simulink model "fboard_xaui"  (Simulink 6.2)
settings: Solver=FixedStepDiscrete  SolverMode=SingleTasking  StartTime=0.0  StopTime=10.0  FixedStep=1  RelTol=1e-3
libraries: xbsIndex_r3 x338, fb_xaui x1, newfft_library x1
(part 2 of 3)

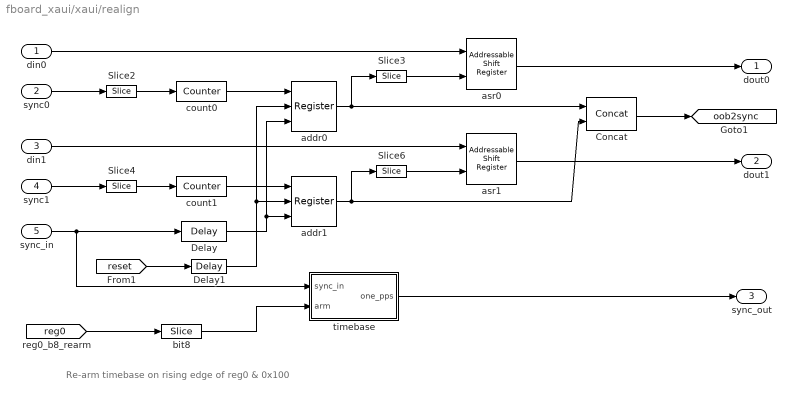
== system fboard_xaui/xaui/realign ==
  note: Re-arm timebase on rising
      | edge of reg0 & 0x100
  din0 : Inport  Port=1  LatchInput=off
  sync0 : Inport  Port=2  LatchInput=off
  din1 : Inport  Port=3  LatchInput=off
  sync1 : Inport  Port=4  LatchInput=off
  sync_in : Inport  Port=5  LatchInput=off
  Concat : xbsIndex_r3/Concat  num_inputs=2  explicit_period=off  period=1  dbl_ovrd=off
  Delay : xbsIndex_r3/Delay  latency=1  reg_retiming=off  explicit_period=off  period=1  en=off  accept_only_valid=off  init_zero=on  dbl_ovrd=off  show_param=off
      settings: xl_area=[1 1 0 0 0 0 0]
  Delay1 : xbsIndex_r3/Delay  latency=1  reg_retiming=off  explicit_period=off  period=1  en=off  accept_only_valid=off  init_zero=on  dbl_ovrd=off  show_param=off
      settings: xl_area=[1 1 0 0 0 0 0]
  Slice2 : xbsIndex_r3/Slice  mode=Lower Bit Location + Width  nbits=1  bit1=0  base1=MSB of Input  bit0=0  base0=LSB of Input  boolean_output=on  explicit_period=off  period=1  dbl_ovrd=off
  Slice3 : xbsIndex_r3/Slice  mode=Lower Bit Location + Width  nbits=6  bit1=0  base1=MSB of Input  bit0=0  base0=LSB of Input  boolean_output=off  explicit_period=off  period=1  dbl_ovrd=off
  Slice4 : xbsIndex_r3/Slice  mode=Lower Bit Location + Width  nbits=1  bit1=0  base1=MSB of Input  bit0=0  base0=LSB of Input  boolean_output=on  explicit_period=off  period=1  dbl_ovrd=off
  Slice6 : xbsIndex_r3/Slice  mode=Lower Bit Location + Width  nbits=6  bit1=0  base1=MSB of Input  bit0=0  base0=LSB of Input  boolean_output=off  explicit_period=off  period=1  dbl_ovrd=off
  addr0 : xbsIndex_r3/Register  init=hex2dec('DEC0')  reg_only_valid=off  explicit_period=off  period=1  rst=on  en=on  out_en=off  dbl_ovrd=off  show_param=on
      settings: xl_area=[3 6 0 0 0 0 0]
  addr1 : xbsIndex_r3/Register  init=hex2dec('DEC0')  reg_only_valid=off  explicit_period=off  period=1  rst=on  en=on  out_en=off  dbl_ovrd=off  show_param=on
      settings: xl_area=[3 6 0 0 0 0 0]
  asr0 : xbsIndex_r3/Addressable Shift Register  infer_latency=on  depth=64  initVector=[0]  explicit_period=off  period=1  accept_only_valid=off  en=off  dbl_ovrd=off  show_param=on  use_rpm=on  gen_core=off
      settings: xl_area=[192 0 0 384 0 0 0]
  asr1 : xbsIndex_r3/Addressable Shift Register  infer_latency=on  depth=64  initVector=[0]  explicit_period=off  period=1  accept_only_valid=off  en=off  dbl_ovrd=off  show_param=on  use_rpm=on  gen_core=off
      settings: xl_area=[192 0 0 384 0 0 0]
  bit8 : xbsIndex_r3/Slice  mode=Lower Bit Location + Width  nbits=1  bit1=12  base1=MSB of Input  bit0=8  base0=LSB of Input  boolean_output=on  explicit_period=off  period=1  dbl_ovrd=off
  count0 : xbsIndex_r3/Counter  cnt_type=Count Limited  n_bits=16  bin_pt=0  arith_type=Unsigned  start_count=0  cnt_to=hex2dec('FFFF')  cnt_by_val=1  operation=Up  explicit_period=off  period=1  load_pin=off  rst=on  en=off  dbl_ovrd=off  show_param=on  use_rpm=on  gen_core=off
      settings: xl_area=[3 6 0 6 0 0 0]
  count1 : xbsIndex_r3/Counter  cnt_type=Count Limited  n_bits=16  bin_pt=0  arith_type=Unsigned  start_count=0  cnt_to=hex2dec('FFFF')  cnt_by_val=1  operation=Up  explicit_period=off  period=1  load_pin=off  rst=on  en=off  dbl_ovrd=off  show_param=on  use_rpm=on  gen_core=off
      settings: xl_area=[3 6 0 6 0 0 0]
  timebase : Subsystem
  dout0 : Outport
  dout1 : Outport  Port=2
  sync_out : Outport  Port=3
  tag scope: oob2sync=global
  wires:
  count0/1 -> addr0/1
  addr0/1 -> Slice3/1, Concat/1
  count1/1 -> addr1/1
  addr1/1 -> Slice6/1, Concat/2
  din0/1 -> asr0/1
  asr0/1 -> dout0/1
  sync0/1 -> Slice2/1
  din1/1 -> asr1/1
  asr1/1 -> dout1/1
  sync1/1 -> Slice4/1
  sync_in/1 -> Delay/1, timebase/1(sync_in)
  timebase/1(one_pps) -> sync_out/1
  bit8/1 -> timebase/2(arm)
  [reg0] -> bit8/1
  Slice2/1 -> count0/1
  Slice4/1 -> count1/1
  Delay/1 -> addr0/3, addr1/3
  Slice3/1 -> asr0/2
  Slice6/1 -> asr1/2
  Concat/1 -> [oob2sync]
  [reset] -> Delay1/1
  Delay1/1 -> addr0/2, addr1/2

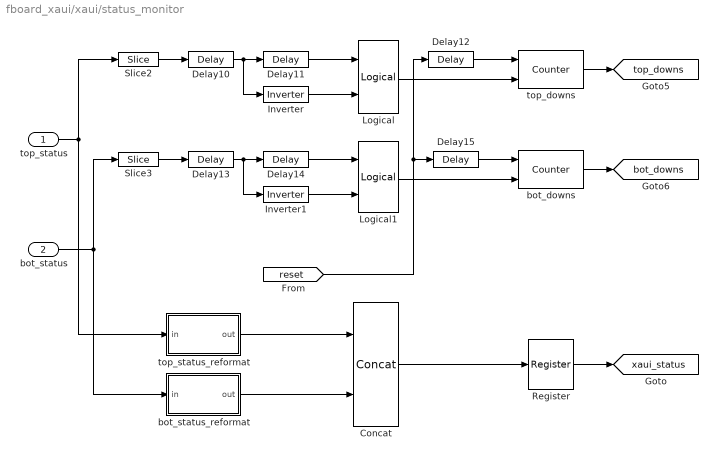
== system fboard_xaui/xaui/status_monitor ==
  top_status : Inport  Port=1  LatchInput=off
  bot_status : Inport  Port=2  LatchInput=off
  Concat : xbsIndex_r3/Concat  num_inputs=2  explicit_period=off  period=1  dbl_ovrd=off
  Delay{10..15} (6 alike) : xbsIndex_r3/Delay  latency=1  reg_retiming=off  explicit_period=off  period=1  en=off  accept_only_valid=off  init_zero=on  dbl_ovrd=off  show_param=off
      settings: xl_area=[0, 0, 0, 0, 0, 0, 0]
  Inverter : xbsIndex_r3/Inverter  latency=0  explicit_period=off  period=1  en=off  dbl_ovrd=off  show_param=off
      settings: xl_area=[0, 0, 0, 0, 0, 0, 0]
  Inverter1 : xbsIndex_r3/Inverter  latency=0  explicit_period=off  period=1  en=off  dbl_ovrd=off  show_param=off
      settings: xl_area=[0, 0, 0, 0, 0, 0, 0]
  Logical : xbsIndex_r3/Logical  logical_function=AND  inputs=2  precision=Full  arith_type=Unsigned  n_bits=8  bin_pt=2  align_bp=on  latency=0  explicit_period=off  period=1  en=off  dbl_ovrd=off  show_param=off
      settings: xl_area=[0, 0, 0, 0, 0, 0, 0]
  Logical1 : xbsIndex_r3/Logical  logical_function=AND  inputs=2  precision=Full  arith_type=Unsigned  n_bits=8  bin_pt=2  align_bp=on  latency=0  explicit_period=off  period=1  en=off  dbl_ovrd=off  show_param=off
      settings: xl_area=[0, 0, 0, 0, 0, 0, 0]
  Register : xbsIndex_r3/Register  init=0  reg_only_valid=off  explicit_period=off  period=1  rst=off  en=off  out_en=off  dbl_ovrd=off  show_param=off
      settings: xl_area=[0, 0, 0, 0, 0, 0, 0]
  Slice2 : xbsIndex_r3/Slice  mode=Lower Bit Location + Width  nbits=1  bit1=12  base1=MSB of Input  bit0=12  base0=LSB of Input  boolean_output=on  explicit_period=off  period=1  dbl_ovrd=off
  Slice3 : xbsIndex_r3/Slice  mode=Lower Bit Location + Width  nbits=1  bit1=12  base1=MSB of Input  bit0=12  base0=LSB of Input  boolean_output=on  explicit_period=off  period=1  dbl_ovrd=off
  bot_downs : xbsIndex_r3/Counter  cnt_type=Free Running  n_bits=32  bin_pt=0  arith_type=Unsigned  start_count=0  cnt_to=Inf  cnt_by_val=1  operation=Up  explicit_period=off  period=1  load_pin=off  rst=on  en=on  dbl_ovrd=off  show_param=off  use_rpm=on  gen_core=off
      settings: xl_area=[0, 0, 0, 0, 0, 0, 0]
  bot_status_reformat : Subsystem
  top_downs : xbsIndex_r3/Counter  cnt_type=Free Running  n_bits=32  bin_pt=0  arith_type=Unsigned  start_count=0  cnt_to=Inf  cnt_by_val=1  operation=Up  explicit_period=off  period=1  load_pin=off  rst=on  en=on  dbl_ovrd=off  show_param=off  use_rpm=on  gen_core=off
      settings: xl_area=[0, 0, 0, 0, 0, 0, 0]
  top_status_reformat : Subsystem
  tag scope: bot_downs=global, top_downs=global, xaui_status=global
  wires:
  top_status/1 -> Slice2/1, top_status_reformat/1(in)
  bot_status/1 -> Slice3/1, bot_status_reformat/1(in)
  top_status_reformat/1(out) -> Concat/1
  bot_status_reformat/1(out) -> Concat/2
  Register/1 -> [xaui_status]
  Concat/1 -> Register/1
  [reset] -> Delay15/1, Delay12/1
  Delay10/1 -> Delay11/1, Inverter/1
  Delay11/1 -> Logical/1
  Inverter/1 -> Logical/2
  Delay12/1 -> top_downs/1
  top_downs/1 -> [top_downs]
  Delay13/1 -> Delay14/1, Inverter1/1
  Delay14/1 -> Logical1/1
  Inverter1/1 -> Logical1/2
  Delay15/1 -> bot_downs/1
  bot_downs/1 -> [bot_downs]
  Logical1/1 -> bot_downs/2
  Logical/1 -> top_downs/2
  Slice2/1 -> Delay10/1
  Slice3/1 -> Delay13/1

== system fboard_xaui/xaui/sync_monitor ==
  top_sync : Inport  Port=1  LatchInput=off
  bot_sync : Inport  Port=2  LatchInput=off
  Delay{4..7} (4 alike) : xbsIndex_r3/Delay  latency=1  reg_retiming=off  explicit_period=off  period=1  en=off  accept_only_valid=off  init_zero=on  dbl_ovrd=off  show_param=off
      settings: xl_area=[0, 0, 0, 0, 0, 0, 0]
  Slice : xbsIndex_r3/Slice  mode=Lower Bit Location + Width  nbits=1  bit1=0  base1=MSB of Input  bit0=0  base0=LSB of Input  boolean_output=on  explicit_period=off  period=1  dbl_ovrd=off
  Slice1 : xbsIndex_r3/Slice  mode=Lower Bit Location + Width  nbits=1  bit1=0  base1=MSB of Input  bit0=0  base0=LSB of Input  boolean_output=on  explicit_period=off  period=1  dbl_ovrd=off
  bot_syncs : xbsIndex_r3/Counter  cnt_type=Free Running  n_bits=32  bin_pt=0  arith_type=Unsigned  start_count=0  cnt_to=Inf  cnt_by_val=1  operation=Up  explicit_period=off  period=1  load_pin=off  rst=on  en=on  dbl_ovrd=off  show_param=off  use_rpm=on  gen_core=off
      settings: xl_area=[0, 0, 0, 0, 0, 0, 0]
  top_syncs : xbsIndex_r3/Counter  cnt_type=Free Running  n_bits=32  bin_pt=0  arith_type=Unsigned  start_count=0  cnt_to=Inf  cnt_by_val=1  operation=Up  explicit_period=off  period=1  load_pin=off  rst=on  en=on  dbl_ovrd=off  show_param=off  use_rpm=on  gen_core=off
      settings: xl_area=[0, 0, 0, 0, 0, 0, 0]
  tag scope: bot_syncs=global, top_syncs=global
  wires:
  bot_sync/1 -> Slice1/1
  Delay4/1 -> top_syncs/1
  Delay5/1 -> bot_syncs/1
  top_syncs/1 -> [top_syncs]
  bot_syncs/1 -> [bot_syncs]
  Delay6/1 -> top_syncs/2
  Delay7/1 -> bot_syncs/2
  top_sync/1 -> Slice/1
  [reset] -> Delay5/1, Delay4/1
  Slice1/1 -> Delay7/1
  Slice/1 -> Delay6/1

== system fboard_xaui/xaui/sync_sel ==
  note: reg0 & 0x30
  top_sync : Inport  Port=1  LatchInput=off
  bot_sync : Inport  Port=2  LatchInput=off
  ext_sync : Inport  Port=3  LatchInput=off
  Delay : xbsIndex_r3/Delay  latency=31  reg_retiming=off  explicit_period=off  period=1  en=off  accept_only_valid=off  init_zero=on  dbl_ovrd=off  show_param=off
      settings: xl_area=[0, 0, 0, 0, 0, 0, 0]
  Mux : xbsIndex_r3/Mux  inputs=4  precision=Full  arith_type="Signed  (2's comp)"  n_bits=8  bin_pt=2  quantization=Truncate  overflow=Wrap  latency=1  explicit_period=off  period=1  en=off  dbl_ovrd=off  show_param=off  mux_type=off  use_rpm=off  gen_core=off
      settings: xl_area=[0, 0, 0, 0, 0, 0, 0]
  Slice1 : xbsIndex_r3/Slice  mode=Lower Bit Location + Width  nbits=1  bit1=0  base1=MSB of Input  bit0=1  base0=LSB of Input  boolean_output=on  explicit_period=off  period=1  dbl_ovrd=off
  Slice4 : xbsIndex_r3/Slice  mode=Lower Bit Location + Width  nbits=1  bit1=0  base1=MSB of Input  bit0=1  base0=LSB of Input  boolean_output=on  explicit_period=off  period=1  dbl_ovrd=off
  b5_b4 : xbsIndex_r3/Slice  mode=Lower Bit Location + Width  nbits=2  bit1=12  base1=MSB of Input  bit0=4  base0=LSB of Input  boolean_output=off  explicit_period=off  period=1  dbl_ovrd=off
  sync_out : Outport
  wires:
  Mux/1 -> Delay/1
  top_sync/1 -> Slice4/1
  bot_sync/1 -> Slice1/1
  Delay/1 -> sync_out/1
  b5_b4/1 -> Mux/1
  [reg0] -> b5_b4/1
  ext_sync/1 -> Mux/4, Mux/5
  Slice4/1 -> Mux/2
  Slice1/1 -> Mux/3

== system fboard_xaui/xaui/uflow_monitor ==
  note: Count rising edges of the rx_empty signals
  top_rx_empty : Inport  Port=1  LatchInput=off
  bot_rx_empty : Inport  Port=2  LatchInput=off
  Concat : xbsIndex_r3/Concat  num_inputs=2  explicit_period=off  period=1  dbl_ovrd=off
  Delay{1,11..12,15} (4 alike) : xbsIndex_r3/Delay  latency=1  reg_retiming=off  explicit_period=off  period=1  en=off  accept_only_valid=off  init_zero=on  dbl_ovrd=off  show_param=off
      settings: xl_area=[0, 0, 0, 0, 0, 0, 0]
  Expression : xbsIndex_r3/Expression  expression=curr & ~prev  precision=Full  arith_type=Unsigned  n_bits=8  bin_pt=2  align_bp=on  latency=0  explicit_period=off  period=1  en=off  dbl_ovrd=off  show_param=off
      settings: xl_area=[0, 0, 0, 0, 0, 0, 0]
  Expression1 : xbsIndex_r3/Expression  expression=curr & ~prev  precision=Full  arith_type=Unsigned  n_bits=8  bin_pt=2  align_bp=on  latency=0  explicit_period=off  period=1  en=off  dbl_ovrd=off  show_param=off
      settings: xl_area=[0, 0, 0, 0, 0, 0, 0]
  bot_uflows : xbsIndex_r3/Counter  cnt_type=Free Running  n_bits=16  bin_pt=0  arith_type=Unsigned  start_count=0  cnt_to=Inf  cnt_by_val=1  operation=Up  explicit_period=off  period=1  load_pin=off  rst=on  en=on  dbl_ovrd=off  show_param=off  use_rpm=on  gen_core=off
      settings: xl_area=[0, 0, 0, 0, 0, 0, 0]
  top_uflows : xbsIndex_r3/Counter  cnt_type=Free Running  n_bits=16  bin_pt=0  arith_type=Unsigned  start_count=0  cnt_to=Inf  cnt_by_val=1  operation=Up  explicit_period=off  period=1  load_pin=off  rst=on  en=on  dbl_ovrd=off  show_param=off  use_rpm=on  gen_core=off
      settings: xl_area=[0, 0, 0, 0, 0, 0, 0]
  tag scope: xaui_uflows=global
  wires:
  [reset] -> Delay15/1, Delay12/1
  Delay12/1 -> top_uflows/1
  top_uflows/1 -> Concat/1
  Delay15/1 -> bot_uflows/1
  bot_uflows/1 -> Concat/2
  Concat/1 -> [xaui_uflows]
  Delay11/1 -> Expression/2
  top_rx_empty/1 -> Delay11/1, Expression/1
  Expression/1 -> top_uflows/2
  Delay1/1 -> Expression1/2
  bot_rx_empty/1 -> Expression1/1, Delay1/1
  Expression1/1 -> bot_uflows/2

== system fboard_xaui/zbt_transpose/dvgen ==
  note: This dvgen block generates a dv signal based on sync_in's rising
      | edge and the value of ds_sel (downsample select), which is taken
      | from a global goto tag.  ds_sel can range from 0 to 7.  The dv
      | signal will be asserted for one cycle every 2^ds_sel cycles starting
      | with the first cycle after sync_out's rising edge.  Note that sync_in
      | may be one or many cycles wide, but it should probably be no
      | wider than 2^ds_sel cycles for typical usage.  sync_out is always
      | one cycle wide (corresponding to the first active cycle of sync_in).
  note: == Example Timing Diagrams ==
      |
      | -------  ds_sel == 0  -------
      | sync_in : .S................
      | sync_out : ....S.............
      | dv : 111111111111111111
      |
      | -------  ds_sel == 1  -------
      | sync_in : .S................
      | sync_out : ....S.............
      | dv : XXXX1.1.1.1.1.1.1.
      |
      | -------  ds_sel == 2  -------
      | sync_in : .SSSS.............
      | sync_out : ....S.............
      | dv : XXXX1...1...1...1.
  note: Only honor new ds_sel value
      | on rising edge of sync_in
  sync_in : Inport  Port=1  LatchInput=off
  Constant2 : xbsIndex_r3/Constant  const=0  equ=P=C  arith_type=Unsigned  n_bits=1  bin_pt=0  opselect=C  inp2=PCIN>>17  opr=+  inp1=P  carry=CIN  iostate=0  explicit_period=on  period=1  dbl_ovrd=off
  Counter : xbsIndex_r3/Counter  cnt_type=Free Running  n_bits=7  bin_pt=0  arith_type=Unsigned  start_count=0  cnt_to=Inf  cnt_by_val=1  operation=Up  explicit_period=off  period=1  load_pin=off  rst=on  en=off  dbl_ovrd=off  show_param=on  use_rpm=on  gen_core=off
      settings: xl_area=[0, 0, 0, 0, 0, 0, 0]
  Delay : xbsIndex_r3/Delay  latency=3  reg_retiming=off  explicit_period=off  period=1  en=off  accept_only_valid=off  init_zero=on  dbl_ovrd=off  show_param=off
      settings: xl_area=[0, 0, 0, 0, 0, 0, 0]
  Mux : xbsIndex_r3/Mux  inputs=8  precision=Full  arith_type="Signed  (2's comp)"  n_bits=8  bin_pt=2  quantization=Truncate  overflow=Wrap  latency=1  explicit_period=off  period=1  en=off  dbl_ovrd=off  show_param=off  mux_type=off  use_rpm=off  gen_core=off
      settings: xl_area=[0, 0, 0, 0, 0, 0, 0]
  Register2 : xbsIndex_r3/Register  init=0  reg_only_valid=off  explicit_period=off  period=1  rst=off  en=on  out_en=off  dbl_ovrd=off  show_param=off
      settings: xl_area=[0, 0, 0, 0, 0, 0, 0]
  Relational : xbsIndex_r3/Relational  mode=a=b  latency=1  explicit_period=off  period=1  en=off  dbl_ovrd=off  show_param=on
      settings: xl_area=[0, 0, 0, 0, 0, 0, 0]
  bit_slicer : Subsystem
  edge_detect : Subsystem  mask(Edge Detector){edge=Rising, polarity=Active High, xin=floor([0.5:0.5:5])*0.08, yin={[-1,-1,1,1,1,1,1,1,1,1],[1,1,-1,-1,-1,-1,-1,-1,-1,-1],[-1,-1,1,1,1,1,-1,-1,-1,-1]}, xout=1-floor([5:-0.5:0.5])*0.08, yout={[-1,-1,1,1,-1,-1,-1,-1,-1,-1],[-1,-1,1,1,-1,-1,-1,-1,-1,-1],[-1,-1,1,1,-1,-1,1,1,-1,-1]}}
      mask prompts: edge "Edge Type"; polarity "Output Polarity"; xin "Input X Positions"; yin "Input Y Positions"; xout "Output X Positions"; yout "Output Y Positions"
      mask help: Output is active for one-cycle after each edge of the specified type (i.e. rising, falling or both).
      mask init:
      | edge_detect_init(gcb,edge,polarity);
      settings: AttributesFormatString=|
      | rising edge
      | active high
      mask Help: Output is active for one-cycle after each edge of the specified type (i.e. rising, falling, or both).  Latency is zero.
      mask StyleString: popup(Rising|Falling|Both),popup(Active High|Active Low),edit,edit,edit,edit
      mask Display:
      | plot(xin,0.5+yin{edge}*0.2)
      | plot(xout,0.5+yout{edge}*0.2*(3-2*polarity))
  sync_out : Outport
  dv : Outport  Port=2
  wires:
  bit_slicer/1(zero) -> Mux/2
  bit_slicer/2(b0_0) -> Mux/3
  bit_slicer/3(b1_0) -> Mux/4
  bit_slicer/4(b2_0) -> Mux/5
  bit_slicer/5(b3_0) -> Mux/6
  bit_slicer/6(b4_0) -> Mux/7
  bit_slicer/7(b5_0) -> Mux/8
  bit_slicer/8(b6_0) -> Mux/9
  Counter/1 -> bit_slicer/1(in)
  Register2/1 -> Mux/1
  Mux/1 -> Relational/2
  sync_in/1 -> edge_detect/1(in)
  Constant2/1 -> Relational/1
  edge_detect/1(out) -> Counter/1, Register2/2, Delay/1
  Delay/1 -> sync_out/1
  Relational/1 -> dv/1
  [ds_sel] -> Register2/1

== system fboard_xaui/bitsel/bitsel_mem/dvgen ==
  note: This dvgen block generates a dv signal based on sync_in's rising
      | edge and the value of ds_sel (downsample select), which is taken
      | from a global goto tag.  ds_sel can range from 0 to 7.  The dv
      | signal will be asserted for one cycle every 2^ds_sel cycles starting
      | with the first cycle after sync_out's rising edge.  Note that sync_in
      | may be one or many cycles wide, but it should probably be no
      | wider than 2^ds_sel cycles for typical usage.  sync_out is always
      | one cycle wide (corresponding to the first active cycle of sync_in).
  note: == Example Timing Diagrams ==
      |
      | -------  ds_sel == 0  -------
      | sync_in : .S................
      | sync_out : ....S.............
      | dv : 111111111111111111
      |
      | -------  ds_sel == 1  -------
      | sync_in : .S................
      | sync_out : ....S.............
      | dv : XXXX1.1.1.1.1.1.1.
      |
      | -------  ds_sel == 2  -------
      | sync_in : .SSSS.............
      | sync_out : ....S.............
      | dv : XXXX1...1...1...1.
  note: Only honor new ds_sel value
      | on rising edge of sync_in
  sync_in : Inport  Port=1  LatchInput=off
  Constant2 : xbsIndex_r3/Constant  const=0  equ=P=C  arith_type=Unsigned  n_bits=1  bin_pt=0  opselect=C  inp2=PCIN>>17  opr=+  inp1=P  carry=CIN  iostate=0  explicit_period=on  period=1  dbl_ovrd=off
  Counter : xbsIndex_r3/Counter  cnt_type=Free Running  n_bits=7  bin_pt=0  arith_type=Unsigned  start_count=0  cnt_to=Inf  cnt_by_val=1  operation=Up  explicit_period=off  period=1  load_pin=off  rst=on  en=off  dbl_ovrd=off  show_param=on  use_rpm=on  gen_core=off
      settings: xl_area=[0, 0, 0, 0, 0, 0, 0]
  Delay : xbsIndex_r3/Delay  latency=3  reg_retiming=off  explicit_period=off  period=1  en=off  accept_only_valid=off  init_zero=on  dbl_ovrd=off  show_param=off
      settings: xl_area=[0, 0, 0, 0, 0, 0, 0]
  Mux : xbsIndex_r3/Mux  inputs=8  precision=Full  arith_type="Signed  (2's comp)"  n_bits=8  bin_pt=2  quantization=Truncate  overflow=Wrap  latency=1  explicit_period=off  period=1  en=off  dbl_ovrd=off  show_param=off  mux_type=off  use_rpm=off  gen_core=off
      settings: xl_area=[0, 0, 0, 0, 0, 0, 0]
  Register2 : xbsIndex_r3/Register  init=0  reg_only_valid=off  explicit_period=off  period=1  rst=off  en=on  out_en=off  dbl_ovrd=off  show_param=off
      settings: xl_area=[0, 0, 0, 0, 0, 0, 0]
  Relational : xbsIndex_r3/Relational  mode=a=b  latency=1  explicit_period=off  period=1  en=off  dbl_ovrd=off  show_param=on
      settings: xl_area=[0, 0, 0, 0, 0, 0, 0]
  bit_slicer : Subsystem
  edge_detect : Subsystem  mask(Edge Detector){edge=Rising, polarity=Active High, xin=floor([0.5:0.5:5])*0.08, yin={[-1,-1,1,1,1,1,1,1,1,1],[1,1,-1,-1,-1,-1,-1,-1,-1,-1],[-1,-1,1,1,1,1,-1,-1,-1,-1]}, xout=1-floor([5:-0.5:0.5])*0.08, yout={[-1,-1,1,1,-1,-1,-1,-1,-1,-1],[-1,-1,1,1,-1,-1,-1,-1,-1,-1],[-1,-1,1,1,-1,-1,1,1,-1,-1]}}
      mask prompts: edge "Edge Type"; polarity "Output Polarity"; xin "Input X Positions"; yin "Input Y Positions"; xout "Output X Positions"; yout "Output Y Positions"
      mask help: Output is active for one-cycle after each edge of the specified type (i.e. rising, falling or both).
      mask init:
      | edge_detect_init(gcb,edge,polarity);
      settings: AttributesFormatString=|
      | rising edge
      | active high
      mask Help: Output is active for one-cycle after each edge of the specified type (i.e. rising, falling, or both).  Latency is zero.
      mask StyleString: popup(Rising|Falling|Both),popup(Active High|Active Low),edit,edit,edit,edit
      mask Display:
      | plot(xin,0.5+yin{edge}*0.2)
      | plot(xout,0.5+yout{edge}*0.2*(3-2*polarity))
  sync_out : Outport
  dv : Outport  Port=2
  wires:
  bit_slicer/1(zero) -> Mux/2
  bit_slicer/2(b0_0) -> Mux/3
  bit_slicer/3(b1_0) -> Mux/4
  bit_slicer/4(b2_0) -> Mux/5
  bit_slicer/5(b3_0) -> Mux/6
  bit_slicer/6(b4_0) -> Mux/7
  bit_slicer/7(b5_0) -> Mux/8
  bit_slicer/8(b6_0) -> Mux/9
  Counter/1 -> bit_slicer/1(in)
  Register2/1 -> Mux/1
  Mux/1 -> Relational/2
  sync_in/1 -> edge_detect/1(in)
  Constant2/1 -> Relational/1
  edge_detect/1(out) -> Counter/1, Register2/2, Delay/1
  Delay/1 -> sync_out/1
  Relational/1 -> dv/1
  [ds_sel] -> Register2/1

== system fboard_xaui/bitsel/bitsel_mem/test_bitsel_mux ==
  sync_in : Inport  Port=1  LatchInput=off
  dv : Inport  Port=2  LatchInput=off
  test_in : Inport  Port=3  LatchInput=off
  chop_en : Inport  Port=4  LatchInput=off
  Counter : xbsIndex_r3/Counter  cnt_type=Free Running  n_bits=13  bin_pt=0  arith_type=Unsigned  start_count=0  cnt_to=Inf  cnt_by_val=1  operation=Up  explicit_period=off  period=1  load_pin=off  rst=on  en=on  dbl_ovrd=off  show_param=off  use_rpm=on  gen_core=off
      settings: xl_area=[0, 0, 0, 0, 0, 0, 0]
  Logical : xbsIndex_r3/Logical  logical_function=AND  inputs=2  precision=Full  arith_type=Unsigned  n_bits=8  bin_pt=2  align_bp=on  latency=0  explicit_period=off  period=1  en=off  dbl_ovrd=off  show_param=off
      settings: xl_area=[0, 0, 0, 0, 0, 0, 0]
  Logical1 : xbsIndex_r3/Logical  logical_function=XOR  inputs=2  precision=Full  arith_type=Unsigned  n_bits=8  bin_pt=2  align_bp=on  latency=0  explicit_period=off  period=1  en=off  dbl_ovrd=off  show_param=off
      settings: xl_area=[0, 0, 0, 0, 0, 0, 0]
  Logical2 : xbsIndex_r3/Logical  logical_function=XNOR  inputs=2  precision=Full  arith_type=Unsigned  n_bits=8  bin_pt=2  align_bp=on  latency=0  explicit_period=off  period=1  en=off  dbl_ovrd=off  show_param=off
      settings: xl_area=[0, 0, 0, 0, 0, 0, 0]
  Mux : xbsIndex_r3/Mux  inputs=2  precision=Full  arith_type="Signed  (2's comp)"  n_bits=8  bin_pt=2  quantization=Truncate  overflow=Wrap  latency=0  explicit_period=off  period=1  en=off  dbl_ovrd=off  show_param=off  mux_type=off  use_rpm=off  gen_core=off
      settings: xl_area=[0, 0, 0, 0, 0, 0, 0]
  Mux1 : xbsIndex_r3/Mux  inputs=2  precision=Full  arith_type="Signed  (2's comp)"  n_bits=8  bin_pt=2  quantization=Truncate  overflow=Wrap  latency=0  explicit_period=off  period=1  en=off  dbl_ovrd=off  show_param=off  mux_type=off  use_rpm=off  gen_core=off
      settings: xl_area=[0, 0, 0, 0, 0, 0, 0]
  Slice : xbsIndex_r3/Slice  mode=Upper Bit Location + Width  nbits=1  bit1=0  base1=MSB of Input  bit0=0  base0=LSB of Input  boolean_output=off  explicit_period=off  period=1  dbl_ovrd=off
  c_to_ri1 : Subsystem  mask(Complex to Real-Imag){n_bits=8, bin_pt=0}
      mask prompts: n_bits "Bit Width"; bin_pt "Binary Point"
      mask help: Outputs real and imaginary components of a complex input.
      mask init:
      | c_to_ri_init(gcb,n_bits,bin_pt);
      settings: AttributesFormatString=8_0 r/i
      mask Help:
      | <pre>
      | Description::
      | 
      | Outputs real and imaginary components of a complex input.
      | Useful for simplifying interconnects.
      | See also: Real-Imag to Complex (ri_to_c)
      | 
      | Mask Parameters::
      | 
      | Bit Width (n_bits): Specifies the width of the real/imaginary components.
      | Assumed equal for both components.
      | 
      | Binary Point (bin_pt): Specifies the binary point location in the real/imaginary components.
      | Assumed equal for both components.
      | </pre>
  ri_to_c : Subsystem  mask(Real-Imag to Complex){}
      mask help: Concatenates real and imaginary inputs into a complex output.
      mask init:
      | ri_to_c_init(gcb);
      mask Help:
      | <pre>
      | Description::
      | 
      | Concatenates a real and imaginary input into a complex output.
      | Useful for simplifying interconnects.
      | See also: Complex to Real-Imag (c_to_ri)
      | 
      | Mask Parameters::
      | 
      | (N/A)
      | </pre>
  test_out : Outport
  wires:
  Counter/1 -> Slice/1
  Slice/1 -> Logical/2
  Logical/1 -> Mux1/1, Mux/1
  c_to_ri1/1(re) -> Mux/2, Logical1/1, Logical2/2
  c_to_ri1/2(im) -> Mux1/2, Logical1/2, Logical2/1
  Mux/1 -> ri_to_c/1(re)
  Mux1/1 -> ri_to_c/2(im)
  chop_en/1 -> Logical/1
  sync_in/1 -> Counter/1
  test_in/1 -> c_to_ri1/1(c)
  ri_to_c/1(c) -> test_out/1
  Logical1/1 -> Mux/3
  Logical2/1 -> Mux1/3
  dv/1 -> Counter/2

== system fboard_xaui/ct4/dvgen/bit_slicer ==
  in : Inport  Port=1  LatchInput=off
  Constant : xbsIndex_r3/Constant  const=0  equ=P=C  arith_type=Unsigned  n_bits=1  bin_pt=0  opselect=C  inp2=PCIN>>17  opr=+  inp1=P  carry=CIN  iostate=0  explicit_period=on  period=1  dbl_ovrd=off
  bit6_0 : xbsIndex_r3/Slice  mode=Lower Bit Location + Width  nbits=7  bit1=0  base1=MSB of Input  bit0=0  base0=LSB of Input  boolean_output=off  explicit_period=off  period=1  dbl_ovrd=off
  bits0_0 : xbsIndex_r3/Slice  mode=Lower Bit Location + Width  nbits=1  bit1=0  base1=MSB of Input  bit0=0  base0=LSB of Input  boolean_output=off  explicit_period=off  period=1  dbl_ovrd=off
  bits1_0 : xbsIndex_r3/Slice  mode=Lower Bit Location + Width  nbits=2  bit1=0  base1=MSB of Input  bit0=0  base0=LSB of Input  boolean_output=off  explicit_period=off  period=1  dbl_ovrd=off
  bits2_0 : xbsIndex_r3/Slice  mode=Lower Bit Location + Width  nbits=3  bit1=0  base1=MSB of Input  bit0=0  base0=LSB of Input  boolean_output=off  explicit_period=off  period=1  dbl_ovrd=off
  bits3_0 : xbsIndex_r3/Slice  mode=Lower Bit Location + Width  nbits=4  bit1=0  base1=MSB of Input  bit0=0  base0=LSB of Input  boolean_output=off  explicit_period=off  period=1  dbl_ovrd=off
  bits4_0 : xbsIndex_r3/Slice  mode=Lower Bit Location + Width  nbits=5  bit1=0  base1=MSB of Input  bit0=0  base0=LSB of Input  boolean_output=off  explicit_period=off  period=1  dbl_ovrd=off
  bits5_0 : xbsIndex_r3/Slice  mode=Lower Bit Location + Width  nbits=6  bit1=0  base1=MSB of Input  bit0=0  base0=LSB of Input  boolean_output=off  explicit_period=off  period=1  dbl_ovrd=off
  zero : Outport
  b0_0 : Outport  Port=2
  b1_0 : Outport  Port=3
  b2_0 : Outport  Port=4
  b3_0 : Outport  Port=5
  b4_0 : Outport  Port=6
  b5_0 : Outport  Port=7
  b6_0 : Outport  Port=8
  wires:
  in/1 -> bits5_0/1, bit6_0/1, bits4_0/1, bits3_0/1, bits2_0/1, bits1_0/1, bits0_0/1
  bits0_0/1 -> b0_0/1
  bits1_0/1 -> b1_0/1
  bits2_0/1 -> b2_0/1
  bits3_0/1 -> b3_0/1
  bits4_0/1 -> b4_0/1
  bits5_0/1 -> b5_0/1
  bit6_0/1 -> b6_0/1
  Constant/1 -> zero/1

== system fboard_xaui/ct4/dvgen/edge_detect ==
  in : Inport  Port=1  LatchInput=off
  Delay : xbsIndex_r3/Delay  latency=1  reg_retiming=off  explicit_period=off  period=1  en=off  accept_only_valid=off  init_zero=on  dbl_ovrd=off  show_param=off
      settings: xl_area=[0, 0, 0, 0, 0, 0, 0]
  Inverter : xbsIndex_r3/Inverter  latency=0  explicit_period=off  period=1  en=off  dbl_ovrd=off  show_param=off
      settings: xl_area=[0, 0, 0, 0, 0, 0, 0]
  edge_op : xbsIndex_r3/Logical  logical_function=NOR  inputs=2  precision=Full  arith_type=Unsigned  n_bits=8  bin_pt=2  align_bp=on  latency=0  explicit_period=off  period=1  en=off  dbl_ovrd=off  show_param=off
      settings: xl_area=[0, 0, 0, 0, 0, 0, 0]
  out : Outport
  wires:
  Delay/1 -> edge_op/2
  in/1 -> Delay/1, Inverter/1
  edge_op/1 -> out/1
  Inverter/1 -> edge_op/1

== system fboard_xaui/downsample/dvgen/bit_slicer ==
  in : Inport  Port=1  LatchInput=off
  Constant : xbsIndex_r3/Constant  const=0  equ=P=C  arith_type=Unsigned  n_bits=1  bin_pt=0  opselect=C  inp2=PCIN>>17  opr=+  inp1=P  carry=CIN  iostate=0  explicit_period=on  period=1  dbl_ovrd=off
  bit6_0 : xbsIndex_r3/Slice  mode=Lower Bit Location + Width  nbits=7  bit1=0  base1=MSB of Input  bit0=0  base0=LSB of Input  boolean_output=off  explicit_period=off  period=1  dbl_ovrd=off
  bits0_0 : xbsIndex_r3/Slice  mode=Lower Bit Location + Width  nbits=1  bit1=0  base1=MSB of Input  bit0=0  base0=LSB of Input  boolean_output=off  explicit_period=off  period=1  dbl_ovrd=off
  bits1_0 : xbsIndex_r3/Slice  mode=Lower Bit Location + Width  nbits=2  bit1=0  base1=MSB of Input  bit0=0  base0=LSB of Input  boolean_output=off  explicit_period=off  period=1  dbl_ovrd=off
  bits2_0 : xbsIndex_r3/Slice  mode=Lower Bit Location + Width  nbits=3  bit1=0  base1=MSB of Input  bit0=0  base0=LSB of Input  boolean_output=off  explicit_period=off  period=1  dbl_ovrd=off
  bits3_0 : xbsIndex_r3/Slice  mode=Lower Bit Location + Width  nbits=4  bit1=0  base1=MSB of Input  bit0=0  base0=LSB of Input  boolean_output=off  explicit_period=off  period=1  dbl_ovrd=off
  bits4_0 : xbsIndex_r3/Slice  mode=Lower Bit Location + Width  nbits=5  bit1=0  base1=MSB of Input  bit0=0  base0=LSB of Input  boolean_output=off  explicit_period=off  period=1  dbl_ovrd=off
  bits5_0 : xbsIndex_r3/Slice  mode=Lower Bit Location + Width  nbits=6  bit1=0  base1=MSB of Input  bit0=0  base0=LSB of Input  boolean_output=off  explicit_period=off  period=1  dbl_ovrd=off
  zero : Outport
  b0_0 : Outport  Port=2
  b1_0 : Outport  Port=3
  b2_0 : Outport  Port=4
  b3_0 : Outport  Port=5
  b4_0 : Outport  Port=6
  b5_0 : Outport  Port=7
  b6_0 : Outport  Port=8
  wires:
  in/1 -> bits5_0/1, bit6_0/1, bits4_0/1, bits3_0/1, bits2_0/1, bits1_0/1, bits0_0/1
  bits0_0/1 -> b0_0/1
  bits1_0/1 -> b1_0/1
  bits2_0/1 -> b2_0/1
  bits3_0/1 -> b3_0/1
  bits4_0/1 -> b4_0/1
  bits5_0/1 -> b5_0/1
  bit6_0/1 -> b6_0/1
  Constant/1 -> zero/1

== system fboard_xaui/downsample/dvgen/edge_detect ==
  in : Inport  Port=1  LatchInput=off
  Delay : xbsIndex_r3/Delay  latency=1  reg_retiming=off  explicit_period=off  period=1  en=off  accept_only_valid=off  init_zero=on  dbl_ovrd=off  show_param=off
      settings: xl_area=[0, 0, 0, 0, 0, 0, 0]
  Inverter : xbsIndex_r3/Inverter  latency=0  explicit_period=off  period=1  en=off  dbl_ovrd=off  show_param=off
      settings: xl_area=[0, 0, 0, 0, 0, 0, 0]
  edge_op : xbsIndex_r3/Logical  logical_function=NOR  inputs=2  precision=Full  arith_type=Unsigned  n_bits=8  bin_pt=2  align_bp=on  latency=0  explicit_period=off  period=1  en=off  dbl_ovrd=off  show_param=off
      settings: xl_area=[0, 0, 0, 0, 0, 0, 0]
  out : Outport
  wires:
  Delay/1 -> edge_op/2
  in/1 -> Delay/1, Inverter/1
  edge_op/1 -> out/1
  Inverter/1 -> edge_op/1

== system fboard_xaui/pfb8/fir8/dvgen ==
  note: This dvgen block generates a dv signal based on sync_in's rising
      | edge and the value of ds_sel (downsample select), which is taken
      | from a global goto tag.  ds_sel can range from 0 to 7.  The dv
      | signal will be asserted for one cycle every 2^ds_sel cycles starting
      | with the first cycle after sync_out's rising edge.  Note that sync_in
      | may be one or many cycles wide, but it should probably be no
      | wider than 2^ds_sel cycles for typical usage.  sync_out is always
      | one cycle wide (corresponding to the first active cycle of sync_in).
  note: == Example Timing Diagrams ==
      |
      | -------  ds_sel == 0  -------
      | sync_in : .S................
      | sync_out : ....S.............
      | dv : 111111111111111111
      |
      | -------  ds_sel == 1  -------
      | sync_in : .S................
      | sync_out : ....S.............
      | dv : XXXX1.1.1.1.1.1.1.
      |
      | -------  ds_sel == 2  -------
      | sync_in : .SSSS.............
      | sync_out : ....S.............
      | dv : XXXX1...1...1...1.
  note: Only honor new ds_sel value
      | on rising edge of sync_in
  sync_in : Inport  Port=1  LatchInput=off
  Constant2 : xbsIndex_r3/Constant  const=0  equ=P=C  arith_type=Unsigned  n_bits=1  bin_pt=0  opselect=C  inp2=PCIN>>17  opr=+  inp1=P  carry=CIN  iostate=0  explicit_period=on  period=1  dbl_ovrd=off
  Counter : xbsIndex_r3/Counter  cnt_type=Free Running  n_bits=7  bin_pt=0  arith_type=Unsigned  start_count=0  cnt_to=Inf  cnt_by_val=1  operation=Up  explicit_period=off  period=1  load_pin=off  rst=on  en=off  dbl_ovrd=off  show_param=on  use_rpm=on  gen_core=off
      settings: xl_area=[0, 0, 0, 0, 0, 0, 0]
  Delay : xbsIndex_r3/Delay  latency=3  reg_retiming=off  explicit_period=off  period=1  en=off  accept_only_valid=off  init_zero=on  dbl_ovrd=off  show_param=off
      settings: xl_area=[0, 0, 0, 0, 0, 0, 0]
  Mux : xbsIndex_r3/Mux  inputs=8  precision=Full  arith_type="Signed  (2's comp)"  n_bits=8  bin_pt=2  quantization=Truncate  overflow=Wrap  latency=1  explicit_period=off  period=1  en=off  dbl_ovrd=off  show_param=off  mux_type=off  use_rpm=off  gen_core=off
      settings: xl_area=[0, 0, 0, 0, 0, 0, 0]
  Register2 : xbsIndex_r3/Register  init=0  reg_only_valid=off  explicit_period=off  period=1  rst=off  en=on  out_en=off  dbl_ovrd=off  show_param=off
      settings: xl_area=[0, 0, 0, 0, 0, 0, 0]
  Relational : xbsIndex_r3/Relational  mode=a=b  latency=1  explicit_period=off  period=1  en=off  dbl_ovrd=off  show_param=on
      settings: xl_area=[0, 0, 0, 0, 0, 0, 0]
  bit_slicer : Subsystem
  edge_detect : Subsystem  mask(Edge Detector){edge=Rising, polarity=Active High, xin=floor([0.5:0.5:5])*0.08, yin={[-1,-1,1,1,1,1,1,1,1,1],[1,1,-1,-1,-1,-1,-1,-1,-1,-1],[-1,-1,1,1,1,1,-1,-1,-1,-1]}, xout=1-floor([5:-0.5:0.5])*0.08, yout={[-1,-1,1,1,-1,-1,-1,-1,-1,-1],[-1,-1,1,1,-1,-1,-1,-1,-1,-1],[-1,-1,1,1,-1,-1,1,1,-1,-1]}}
      mask prompts: edge "Edge Type"; polarity "Output Polarity"; xin "Input X Positions"; yin "Input Y Positions"; xout "Output X Positions"; yout "Output Y Positions"
      mask help: Output is active for one-cycle after each edge of the specified type (i.e. rising, falling or both).
      mask init:
      | edge_detect_init(gcb,edge,polarity);
      settings: AttributesFormatString=|
      | rising edge
      | active high
      mask Help: Output is active for one-cycle after each edge of the specified type (i.e. rising, falling, or both).  Latency is zero.
      mask StyleString: popup(Rising|Falling|Both),popup(Active High|Active Low),edit,edit,edit,edit
      mask Display:
      | plot(xin,0.5+yin{edge}*0.2)
      | plot(xout,0.5+yout{edge}*0.2*(3-2*polarity))
  sync_out : Outport
  dv : Outport  Port=2
  wires:
  bit_slicer/1(zero) -> Mux/2
  bit_slicer/2(b0_0) -> Mux/3
  bit_slicer/3(b1_0) -> Mux/4
  bit_slicer/4(b2_0) -> Mux/5
  bit_slicer/5(b3_0) -> Mux/6
  bit_slicer/6(b4_0) -> Mux/7
  bit_slicer/7(b5_0) -> Mux/8
  bit_slicer/8(b6_0) -> Mux/9
  Counter/1 -> bit_slicer/1(in)
  Register2/1 -> Mux/1
  Mux/1 -> Relational/2
  sync_in/1 -> edge_detect/1(in)
  Constant2/1 -> Relational/1
  edge_detect/1(out) -> Counter/1, Register2/2, Delay/1
  Delay/1 -> sync_out/1
  Relational/1 -> dv/1
  [ds_sel] -> Register2/1

== system fboard_xaui/pfb8/fir8/pfb_fir_0 ==
  pol1_in : Inport  Port=1  LatchInput=off
  pol2_in : Inport  Port=2  LatchInput=off
  sync_in : Inport  Port=3  LatchInput=off
  dv : Inport  Port=4  LatchInput=off
  pfb_fir_dv : xbsIndex_r3/Black Box  init_code=pfb_fir_dv_config  sim_method=Inactive  show_param=off
      settings: xl_area=[0, 0, 0, 0, 0, 0, 0]
  pol1_out : Outport
  pol2_out : Outport  Port=2
  sync_out : Outport  Port=3
  wires:
  pol1_in/1 -> pfb_fir_dv/1
  pfb_fir_dv/1 -> pol1_out/1
  pol2_in/1 -> pfb_fir_dv/2
  pfb_fir_dv/2 -> pol2_out/1
  sync_in/1 -> pfb_fir_dv/3
  pfb_fir_dv/3 -> sync_out/1
  dv/1 -> pfb_fir_dv/4

== system fboard_xaui/pfb8/fir8/pfb_fir_1 ==
  pol1_in : Inport  Port=1  LatchInput=off
  pol2_in : Inport  Port=2  LatchInput=off
  sync_in : Inport  Port=3  LatchInput=off
  dv : Inport  Port=4  LatchInput=off
  pfb_fir_dv : xbsIndex_r3/Black Box  init_code=pfb_fir_dv_config  sim_method=Inactive  show_param=off
      settings: xl_area=[0, 0, 0, 0, 0, 0, 0]
  pol1_out : Outport
  pol2_out : Outport  Port=2
  sync_out : Outport  Port=3
  wires:
  pol1_in/1 -> pfb_fir_dv/1
  pfb_fir_dv/1 -> pol1_out/1
  pol2_in/1 -> pfb_fir_dv/2
  pfb_fir_dv/2 -> pol2_out/1
  sync_in/1 -> pfb_fir_dv/3
  pfb_fir_dv/3 -> sync_out/1
  dv/1 -> pfb_fir_dv/4

== system fboard_xaui/pfb8/fir8/pfb_fir_2 ==
  pol1_in : Inport  Port=1  LatchInput=off
  pol2_in : Inport  Port=2  LatchInput=off
  sync_in : Inport  Port=3  LatchInput=off
  dv : Inport  Port=4  LatchInput=off
  pfb_fir_dv : xbsIndex_r3/Black Box  init_code=pfb_fir_dv_config  sim_method=Inactive  show_param=off
      settings: xl_area=[0, 0, 0, 0, 0, 0, 0]
  pol1_out : Outport
  pol2_out : Outport  Port=2
  sync_out : Outport  Port=3
  wires:
  pol1_in/1 -> pfb_fir_dv/1
  pfb_fir_dv/1 -> pol1_out/1
  pol2_in/1 -> pfb_fir_dv/2
  pfb_fir_dv/2 -> pol2_out/1
  sync_in/1 -> pfb_fir_dv/3
  pfb_fir_dv/3 -> sync_out/1
  dv/1 -> pfb_fir_dv/4

== system fboard_xaui/pfb8/fir8/pfb_fir_3 ==
  pol1_in : Inport  Port=1  LatchInput=off
  pol2_in : Inport  Port=2  LatchInput=off
  sync_in : Inport  Port=3  LatchInput=off
  dv : Inport  Port=4  LatchInput=off
  pfb_fir_dv : xbsIndex_r3/Black Box  init_code=pfb_fir_dv_config  sim_method=Inactive  show_param=off
      settings: xl_area=[0, 0, 0, 0, 0, 0, 0]
  pol1_out : Outport
  pol2_out : Outport  Port=2
  sync_out : Outport  Port=3
  wires:
  pol1_in/1 -> pfb_fir_dv/1
  pfb_fir_dv/1 -> pol1_out/1
  pol2_in/1 -> pfb_fir_dv/2
  pfb_fir_dv/2 -> pol2_out/1
  sync_in/1 -> pfb_fir_dv/3
  pfb_fir_dv/3 -> sync_out/1
  dv/1 -> pfb_fir_dv/4

== system fboard_xaui/pfb8/pfb_fft8/dvgen ==
  note: This dvgen block generates a dv signal based on sync_in's rising
      | edge and the value of ds_sel (downsample select), which is taken
      | from a global goto tag.  ds_sel can range from 0 to 7.  The dv
      | signal will be asserted for one cycle every 2^ds_sel cycles starting
      | with the first cycle after sync_out's rising edge.  Note that sync_in
      | may be one or many cycles wide, but it should probably be no
      | wider than 2^ds_sel cycles for typical usage.  sync_out is always
      | one cycle wide (corresponding to the first active cycle of sync_in).
  note: == Example Timing Diagrams ==
      |
      | -------  ds_sel == 0  -------
      | sync_in : .S................
      | sync_out : ....S.............
      | dv : 111111111111111111
      |
      | -------  ds_sel == 1  -------
      | sync_in : .S................
      | sync_out : ....S.............
      | dv : XXXX1.1.1.1.1.1.1.
      |
      | -------  ds_sel == 2  -------
      | sync_in : .SSSS.............
      | sync_out : ....S.............
      | dv : XXXX1...1...1...1.
  note: Only honor new ds_sel value
      | on rising edge of sync_in
  sync_in : Inport  Port=1  LatchInput=off
  Constant2 : xbsIndex_r3/Constant  const=0  equ=P=C  arith_type=Unsigned  n_bits=1  bin_pt=0  opselect=C  inp2=PCIN>>17  opr=+  inp1=P  carry=CIN  iostate=0  explicit_period=on  period=1  dbl_ovrd=off
  Counter : xbsIndex_r3/Counter  cnt_type=Free Running  n_bits=7  bin_pt=0  arith_type=Unsigned  start_count=0  cnt_to=Inf  cnt_by_val=1  operation=Up  explicit_period=off  period=1  load_pin=off  rst=on  en=off  dbl_ovrd=off  show_param=on  use_rpm=on  gen_core=off
      settings: xl_area=[0, 0, 0, 0, 0, 0, 0]
  Delay : xbsIndex_r3/Delay  latency=3  reg_retiming=off  explicit_period=off  period=1  en=off  accept_only_valid=off  init_zero=on  dbl_ovrd=off  show_param=off
      settings: xl_area=[0, 0, 0, 0, 0, 0, 0]
  Mux : xbsIndex_r3/Mux  inputs=8  precision=Full  arith_type="Signed  (2's comp)"  n_bits=8  bin_pt=2  quantization=Truncate  overflow=Wrap  latency=1  explicit_period=off  period=1  en=off  dbl_ovrd=off  show_param=off  mux_type=off  use_rpm=off  gen_core=off
      settings: xl_area=[0, 0, 0, 0, 0, 0, 0]
  Register2 : xbsIndex_r3/Register  init=0  reg_only_valid=off  explicit_period=off  period=1  rst=off  en=on  out_en=off  dbl_ovrd=off  show_param=off
      settings: xl_area=[0, 0, 0, 0, 0, 0, 0]
  Relational : xbsIndex_r3/Relational  mode=a=b  latency=1  explicit_period=off  period=1  en=off  dbl_ovrd=off  show_param=on
      settings: xl_area=[0, 0, 0, 0, 0, 0, 0]
  bit_slicer : Subsystem
  edge_detect : Subsystem  mask(Edge Detector){edge=Rising, polarity=Active High, xin=floor([0.5:0.5:5])*0.08, yin={[-1,-1,1,1,1,1,1,1,1,1],[1,1,-1,-1,-1,-1,-1,-1,-1,-1],[-1,-1,1,1,1,1,-1,-1,-1,-1]}, xout=1-floor([5:-0.5:0.5])*0.08, yout={[-1,-1,1,1,-1,-1,-1,-1,-1,-1],[-1,-1,1,1,-1,-1,-1,-1,-1,-1],[-1,-1,1,1,-1,-1,1,1,-1,-1]}}
      mask prompts: edge "Edge Type"; polarity "Output Polarity"; xin "Input X Positions"; yin "Input Y Positions"; xout "Output X Positions"; yout "Output Y Positions"
      mask help: Output is active for one-cycle after each edge of the specified type (i.e. rising, falling or both).
      mask init:
      | edge_detect_init(gcb,edge,polarity);
      settings: AttributesFormatString=|
      | rising edge
      | active high
      mask Help: Output is active for one-cycle after each edge of the specified type (i.e. rising, falling, or both).  Latency is zero.
      mask StyleString: popup(Rising|Falling|Both),popup(Active High|Active Low),edit,edit,edit,edit
      mask Display:
      | plot(xin,0.5+yin{edge}*0.2)
      | plot(xout,0.5+yout{edge}*0.2*(3-2*polarity))
  sync_out : Outport
  dv : Outport  Port=2
  wires:
  bit_slicer/1(zero) -> Mux/2
  bit_slicer/2(b0_0) -> Mux/3
  bit_slicer/3(b1_0) -> Mux/4
  bit_slicer/4(b2_0) -> Mux/5
  bit_slicer/5(b3_0) -> Mux/6
  bit_slicer/6(b4_0) -> Mux/7
  bit_slicer/7(b5_0) -> Mux/8
  bit_slicer/8(b6_0) -> Mux/9
  Counter/1 -> bit_slicer/1(in)
  Register2/1 -> Mux/1
  Mux/1 -> Relational/2
  sync_in/1 -> edge_detect/1(in)
  Constant2/1 -> Relational/1
  edge_detect/1(out) -> Counter/1, Register2/2, Delay/1
  Delay/1 -> sync_out/1
  Relational/1 -> dv/1
  [ds_sel] -> Register2/1

== system fboard_xaui/pfb8/pfb_fft8/quadplex_fft_0 ==
  in0 : Inport  Port=1  LatchInput=off
  in1 : Inport  Port=2  LatchInput=off
  in2 : Inport  Port=3  LatchInput=off
  in3 : Inport  Port=4  LatchInput=off
  sync_in : Inport  Port=5  LatchInput=off
  dv : Inport  Port=6  LatchInput=off
  pfb_fft : xbsIndex_r3/Black Box  init_code=pfb_fft_dv_config  sim_method=Inactive  show_param=off
      settings: xl_area=[0, 0, 0, 0, 0, 0, 0]
  out0 : Outport
  out1 : Outport  Port=2
  out2 : Outport  Port=3
  out3 : Outport  Port=4
  sync_out : Outport  Port=5
  wires:
  in0/1 -> pfb_fft/1
  pfb_fft/1 -> out0/1
  in1/1 -> pfb_fft/2
  pfb_fft/2 -> out1/1
  in2/1 -> pfb_fft/3
  pfb_fft/3 -> out2/1
  in3/1 -> pfb_fft/4
  pfb_fft/4 -> out3/1
  sync_in/1 -> pfb_fft/5
  pfb_fft/5 -> sync_out/1
  dv/1 -> pfb_fft/6

== system fboard_xaui/pfb8/pfb_fft8/quadplex_fft_1 ==
  in0 : Inport  Port=1  LatchInput=off
  in1 : Inport  Port=2  LatchInput=off
  in2 : Inport  Port=3  LatchInput=off
  in3 : Inport  Port=4  LatchInput=off
  sync_in : Inport  Port=5  LatchInput=off
  dv : Inport  Port=6  LatchInput=off
  pfb_fft : xbsIndex_r3/Black Box  init_code=pfb_fft_dv_config  sim_method=Inactive  show_param=off
      settings: xl_area=[0, 0, 0, 0, 0, 0, 0]
  out0 : Outport
  out1 : Outport  Port=2
  out2 : Outport  Port=3
  out3 : Outport  Port=4
  sync_out : Outport  Port=5
  wires:
  in0/1 -> pfb_fft/1
  pfb_fft/1 -> out0/1
  in1/1 -> pfb_fft/2
  pfb_fft/2 -> out1/1
  in2/1 -> pfb_fft/3
  pfb_fft/3 -> out2/1
  in3/1 -> pfb_fft/4
  pfb_fft/4 -> out3/1
  sync_in/1 -> pfb_fft/5
  pfb_fft/5 -> sync_out/1
  dv/1 -> pfb_fft/6

== system fboard_xaui/xaui/llc/falling_edge ==
  in : Inport  Port=1  LatchInput=off
  Delay : xbsIndex_r3/Delay  latency=1  reg_retiming=off  explicit_period=off  period=1  en=off  accept_only_valid=off  init_zero=on  dbl_ovrd=off  show_param=off
      settings: xl_area=[0, 0, 0, 0, 0, 0, 0]
  Expression : xbsIndex_r3/Expression  expression=~curr & prev  precision=Full  arith_type=Unsigned  n_bits=8  bin_pt=2  align_bp=on  latency=0  explicit_period=off  period=1  en=off  dbl_ovrd=off  show_param=off
      settings: xl_area=[0, 0, 0, 0, 0, 0, 0]
  out : Outport
  wires:
  Delay/1 -> Expression/2
  in/1 -> Expression/1, Delay/1
  Expression/1 -> out/1

== system fboard_xaui/xaui/llc/rising_edge ==
  in : Inport  Port=1  LatchInput=off
  Delay : xbsIndex_r3/Delay  latency=1  reg_retiming=off  explicit_period=off  period=1  en=off  accept_only_valid=off  init_zero=on  dbl_ovrd=off  show_param=off
      settings: xl_area=[0, 0, 0, 0, 0, 0, 0]
  Expression : xbsIndex_r3/Expression  expression=curr & ~prev  precision=Full  arith_type=Unsigned  n_bits=8  bin_pt=2  align_bp=on  latency=0  explicit_period=off  period=1  en=off  dbl_ovrd=off  show_param=off
      settings: xl_area=[0, 0, 0, 0, 0, 0, 0]
  out : Outport
  wires:
  Delay/1 -> Expression/2
  in/1 -> Expression/1, Delay/1
  Expression/1 -> out/1

== system fboard_xaui/xaui/realign/timebase ==
  sync_in : Inport  Port=1  LatchInput=off
  arm : Inport  Port=2  LatchInput=off
  Terminator : Terminator
  Terminator2 : Terminator
  Terminator4 : Terminator
  armed_trigger : newfft_library/Utility/armed_trigger  hidden=0
      link override Constant2: equ=P=C
  master_timebase : Subsystem
  one_pps : Outport
  tag scope: mcount=global, one_pps=global, one_ppt=global, time=global
  wires:
  master_timebase/1(master) -> [mcount]
  master_timebase/2(time) -> [time]
  master_timebase/4(one_ppt) -> [one_ppt]
  master_timebase/3(one_pps) -> [one_pps]
  sync_in/1 -> armed_trigger/2
  arm/1 -> armed_trigger/1
  [one_pps] -> one_pps/1
  [mcount] -> Terminator/1
  [time] -> Terminator2/1
  [one_ppt] -> Terminator4/1
  armed_trigger/1 -> master_timebase/1(rst)

== system fboard_xaui/xaui/status_monitor/bot_status_reformat ==
  in : Inport  Port=1  LatchInput=off
  Concat : xbsIndex_r3/Concat  num_inputs=4  explicit_period=off  period=1  dbl_ovrd=off
  aligned : xbsIndex_r3/Slice  mode=Lower Bit Location + Width  nbits=1  bit1=12  base1=MSB of Input  bit0=10  base0=LSB of Input  boolean_output=off  explicit_period=off  period=1  dbl_ovrd=off
  four_bits{1..4} (4 alike) : xbsIndex_r3/Convert  arith_type=Unsigned  n_bits=4  bin_pt=0  quantization=Truncate  overflow=Wrap  latency=0  explicit_period=off  period=1  dbl_ovrd=off  show_param=off  inserted_by_tool=off  pipeline=off
      settings: xl_area=[0, 0, 0, 0, 0, 0, 0]
  fsm : xbsIndex_r3/Slice  mode=Lower Bit Location + Width  nbits=4  bit1=12  base1=MSB of Input  bit0=0  base0=LSB of Input  boolean_output=off  explicit_period=off  period=1  dbl_ovrd=off
  link : xbsIndex_r3/Slice  mode=Lower Bit Location + Width  nbits=1  bit1=12  base1=MSB of Input  bit0=12  base0=LSB of Input  boolean_output=off  explicit_period=off  period=1  dbl_ovrd=off
  syncs : xbsIndex_r3/Slice  mode=Lower Bit Location + Width  nbits=4  bit1=12  base1=MSB of Input  bit0=6  base0=LSB of Input  boolean_output=off  explicit_period=off  period=1  dbl_ovrd=off
  out : Outport
  wires:
  in/1 -> syncs/1, fsm/1, aligned/1, link/1
  Concat/1 -> out/1
  four_bits4/1 -> Concat/4
  four_bits3/1 -> Concat/3
  four_bits2/1 -> Concat/2
  four_bits1/1 -> Concat/1
  fsm/1 -> four_bits4/1
  syncs/1 -> four_bits3/1
  aligned/1 -> four_bits2/1
  link/1 -> four_bits1/1

== system fboard_xaui/xaui/status_monitor/top_status_reformat ==
  in : Inport  Port=1  LatchInput=off
  Concat : xbsIndex_r3/Concat  num_inputs=4  explicit_period=off  period=1  dbl_ovrd=off
  aligned : xbsIndex_r3/Slice  mode=Lower Bit Location + Width  nbits=1  bit1=12  base1=MSB of Input  bit0=10  base0=LSB of Input  boolean_output=off  explicit_period=off  period=1  dbl_ovrd=off
  four_bits{1..4} (4 alike) : xbsIndex_r3/Convert  arith_type=Unsigned  n_bits=4  bin_pt=0  quantization=Truncate  overflow=Wrap  latency=0  explicit_period=off  period=1  dbl_ovrd=off  show_param=off  inserted_by_tool=off  pipeline=off
      settings: xl_area=[0, 0, 0, 0, 0, 0, 0]
  fsm : xbsIndex_r3/Slice  mode=Lower Bit Location + Width  nbits=4  bit1=12  base1=MSB of Input  bit0=0  base0=LSB of Input  boolean_output=off  explicit_period=off  period=1  dbl_ovrd=off
  link : xbsIndex_r3/Slice  mode=Lower Bit Location + Width  nbits=1  bit1=12  base1=MSB of Input  bit0=12  base0=LSB of Input  boolean_output=off  explicit_period=off  period=1  dbl_ovrd=off
  syncs : xbsIndex_r3/Slice  mode=Lower Bit Location + Width  nbits=4  bit1=12  base1=MSB of Input  bit0=6  base0=LSB of Input  boolean_output=off  explicit_period=off  period=1  dbl_ovrd=off
  out : Outport
  wires:
  link/1 -> four_bits1/1
  aligned/1 -> four_bits2/1
  syncs/1 -> four_bits3/1
  fsm/1 -> four_bits4/1
  four_bits1/1 -> Concat/1
  four_bits2/1 -> Concat/2
  four_bits3/1 -> Concat/3
  four_bits4/1 -> Concat/4
  Concat/1 -> out/1
  in/1 -> link/1, aligned/1, fsm/1, syncs/1
